simulink model "Virtual_Exhaust_Aftertreatment_Controller_PRT"  (R2016b)
settings: Solver=FixedStepAuto  StartTime=0.0  StopTime=inf  FixedStep=VirtExhATCtrlr.tiSimnTiStep_C  RelTol=1e-3  SampleTimeConstraint=STIndependent  EnableMultiTasking=on
undefined symbols (not defined in the file or in its folder): CAL, SOUIT, T3LIMCL_COEOM_MSK_SY, T3LimCL_stMskEOM1_C, T3LimCL_stMskEOM2_C, T3LimCL_stMskEOM3_C, VirtExhATCtrlr_numHrznSize_CA
libraries: simulink x4
(part 1 of 5)
settings Model: Creator=m01wolf  LastModifiedBy=bunver
settings DataIOCC: SaveFormat=StructureWithTime  SaveOutput=off  DSMLogging=off  VisualizeSimOutput=off  SaveTime=off  StateSaveName=Results  SignalLoggingName=Results
settings OptimizationCC: BlockReduction=off  ConditionallyExecuteInputs=off  LifeSpan=inf
settings DebuggingCC: AllowSymbolicDim=off  SFUnexpectedBacktrackingDiag=warning  SFNoUnconditionalDefaultTransitionDiag=warning  SFExecutionAtInitializationDiag=none
settings ModelReferenceCC: ModelReferenceNumInstancesAllowed=Single  PropagateSignalLabelsOutOfModel=off
settings GRTTargetCC: TargetLangStandard=C89/C90 (ANSI)
settings ConfigComp: CovMetricSettings=dw  CovHtmlReporting=on  CovSaveCumulativeToWorkspaceVar=on  CovSaveSingleToWorkspaceVar=on  CovExternalEMLEnable=off

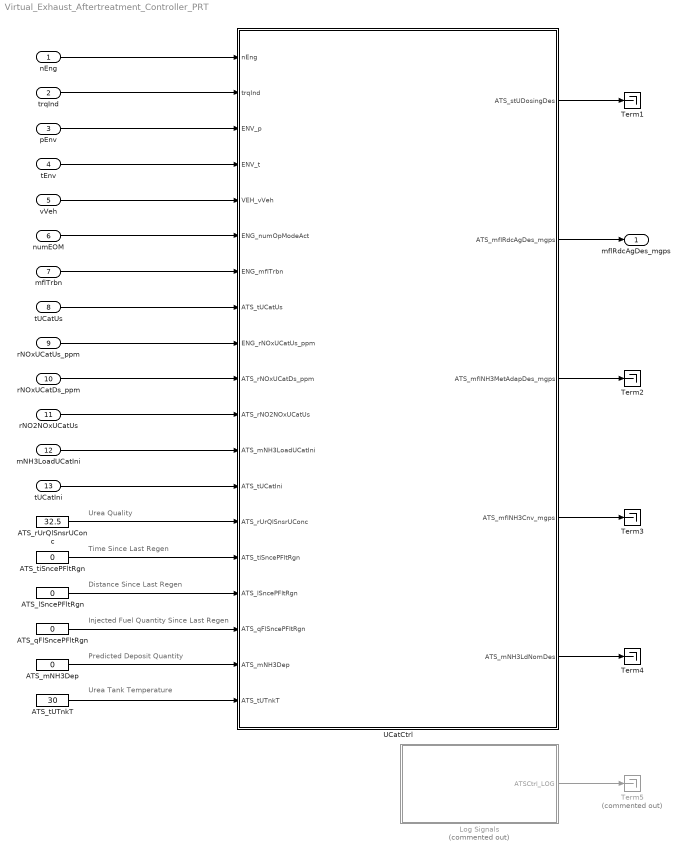
== system Virtual_Exhaust_Aftertreatment_Controller_PRT ==
  note: Urea Quality
  note: Time Since Last Regen
  note: Distance Since Last Regen
  note: Urea Tank Temperature
  note: Predicted Deposit Quantity
  note: Injected Fuel Quantity Since Last Regen
  nEng : Inport  PortDimensions=VirtExhATCtrlr_numHrznSize_CA
  trqInd : Inport  Port=2  PortDimensions=VirtExhATCtrlr_numHrznSize_CA
  "pEnv  " : Inport  Port=3  OutDataTypeStr=double
  "tEnv  " : Inport  Port=4  OutDataTypeStr=double
  vVeh : Inport  Port=5  OutDataTypeStr=double  PortDimensions=VirtExhATCtrlr_numHrznSize_CA
  numEOM : Inport  Port=6  PortDimensions=VirtExhATCtrlr_numHrznSize_CA
  mflTrbn : Inport  Port=7  PortDimensions=VirtExhATCtrlr_numHrznSize_CA
  tUCatUs : Inport  Port=8  PortDimensions=VirtExhATCtrlr_numHrznSize_CA
  rNOxUCatUs_ppm : Inport  Port=9  PortDimensions=VirtExhATCtrlr_numHrznSize_CA
  rNOxUCatDs_ppm : Inport  Port=10  PortDimensions=VirtExhATCtrlr_numHrznSize_CA
  rNO2NOxUCatUs : Inport  Port=11  PortDimensions=VirtExhATCtrlr_numHrznSize_CA
  mNH3LoadUCatIni : Inport  Port=12
  tUCatIni : Inport  Port=13
  ATS_lSncePFltRgn : Constant  Value=0  SampleTime=-1
  ATS_mNH3Dep : Constant  Value=0  SampleTime=-1
  ATS_qFlSncePFltRgn : Constant  Value=0  SampleTime=-1
  ATS_rUrQlSnsrUConc : Constant  Value=32.5  SampleTime=-1
  ATS_tUTnkT : Constant  Value=30  SampleTime=-1
  ATS_tiSncePFltRgn : Constant  Value=0  SampleTime=-1
  Log Signals : Subsystem  Commented=on
  Term{1..4} (4 alike) : Terminator
  Term5 : Terminator  Commented=on
  UCatCtrl : Subsystem
  mflRdcAgDes_mgps : Outport
  wires:
  UCatCtrl/1(ATS_stUDosingDes) -> Term1/1
  UCatCtrl/2(ATS_mflRdcAgDes_mgps) -> mflRdcAgDes_mgps/1
  UCatCtrl/3(ATS_mflNH3MetAdapDes_mgps) -> Term2/1
  UCatCtrl/4(ATS_mflNH3Cnv_mgps) -> Term3/1
  UCatCtrl/5(ATS_mNH3LdNomDes) -> Term4/1
  Log Signals/1(ATSCtrl_LOG) -> Term5/1
  nEng/1 -> UCatCtrl/1(nEng)
  trqInd/1 -> UCatCtrl/2(trqInd)
  "pEnv  "/1 -> UCatCtrl/3(ENV_p)
  "tEnv  "/1 -> UCatCtrl/4(ENV_t)
  vVeh/1 -> UCatCtrl/5(VEH_vVeh)
  numEOM/1 -> UCatCtrl/6(ENG_numOpModeAct)
  mflTrbn/1 -> UCatCtrl/7(ENG_mflTrbn)
  tUCatUs/1 -> UCatCtrl/8(ATS_tUCatUs)
  rNOxUCatUs_ppm/1 -> UCatCtrl/9(ENG_rNOxUCatUs_ppm)
  rNOxUCatDs_ppm/1 -> UCatCtrl/10(ATS_rNOxUCatDs_ppm)
  rNO2NOxUCatUs/1 -> UCatCtrl/11(ATS_rNO2NOxUCatUs)
  mNH3LoadUCatIni/1 -> UCatCtrl/12(ATS_mNH3LoadUCatIni)
  tUCatIni/1 -> UCatCtrl/13(ATS_tUCatIni)
  ATS_tiSncePFltRgn/1 -> UCatCtrl/15(ATS_tiSncePFltRgn)
  ATS_qFlSncePFltRgn/1 -> UCatCtrl/17(ATS_qFlSncePFltRgn)
  ATS_tUTnkT/1 -> UCatCtrl/19(ATS_tUTnkT)
  ATS_mNH3Dep/1 -> UCatCtrl/18(ATS_mNH3Dep)
  ATS_lSncePFltRgn/1 -> UCatCtrl/16(ATS_lSncePFltRgn)
  ATS_rUrQlSnsrUConc/1 -> UCatCtrl/14(ATS_rUrQlSnsrUConc)

== system Virtual_Exhaust_Aftertreatment_Controller_PRT/Log Signals ==
  BusCreator1 : BusCreator  Inputs=23
  ATSCtrl_LOG : Outport
  wires:
  BusCreator1/1 -> ATSCtrl_LOG/1  "ATSCtrl_LOG_BUS"
  [ATS_etaEstNOxCnvUCat] -> BusCreator1/1
  [ATS_facEstEfcUCatAge] -> BusCreator1/2
  [ATS_mEstNH3LoadUCat] -> BusCreator1/3
  [ATS_mflEstNH3OxiUCatUs_mgps] -> BusCreator1/4
  [ATS_rEstNOxUCatDs_ppm] -> BusCreator1/5
  [ATS_tEstUCatAvrg] -> BusCreator1/6
  [ATS_mflNH3OxiUCatUs_mgps] -> BusCreator1/7
  [DepLimCor_facNH3MaxCor] -> BusCreator1/8
  [SCRLdG_dmNH3Max] -> BusCreator1/9
  [ATS_facNOxCtl] -> BusCreator1/10
  [ATS_facQtyAdap] -> BusCreator1/11
  [ATS_mNH3LdNom] -> BusCreator1/12
  [ATS_mNH3LoadUCatRst] -> BusCreator1/13
  [ATS_mflNH3Cnv_mgps] -> BusCreator1/14
  [ATS_mflNH3CurrEfc_mgps] -> BusCreator1/15
  [ATS_mflNH3DpstLmt_mgps] -> BusCreator1/16
  [ATS_mflNH3MetAdapDes_mgps] -> BusCreator1/17
  [ATS_mflNH3PreCtl_mgps] -> BusCreator1/18
  [ATS_mflNH3_mgps] -> BusCreator1/19
  [ATS_mflNOxUs_mgps] -> BusCreator1/20
  [ATS_stNH3LoadUCatRst] -> BusCreator1/21
  [ATS_stUDosing] -> BusCreator1/22
  [EvpMod_tUCatUsT] -> BusCreator1/23

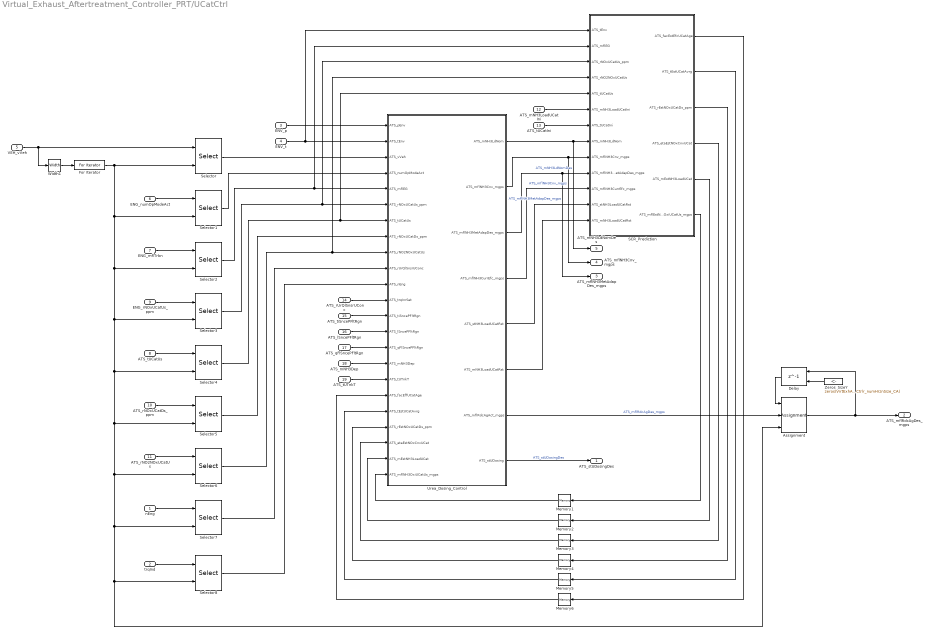
== system Virtual_Exhaust_Aftertreatment_Controller_PRT/UCatCtrl ==
  nEng : Inport
  trqInd : Inport  Port=2
  ENV_p : Inport  Port=3
  ENV_t : Inport  Port=4
  VEH_vVeh : Inport  Port=5
  ENG_numOpModeAct : Inport  Port=6
  ENG_mflTrbn : Inport  Port=7
  ATS_tUCatUs : Inport  Port=8
  ENG_rNOxUCatUs_ppm : Inport  Port=9
  ATS_rNOxUCatDs_ppm : Inport  Port=10
  ATS_rNO2NOxUCatUs : Inport  Port=11
  ATS_mNH3LoadUCatIni : Inport  Port=12
  ATS_tUCatIni : Inport  Port=13
  ATS_rUrQlSnsrUConc : Inport  Port=14
  ATS_tiSncePFltRgn : Inport  Port=15
  ATS_lSncePFltRgn : Inport  Port=16
  ATS_qFlSncePFltRgn : Inport  Port=17
  ATS_mNH3Dep : Inport  Port=18
  ATS_tUTnkT : Inport  Port=19
  Assignment : Assignment  DiagnosticForDimensions=Warning  IndexOptions=Starting index (port)  Indices=1  OutputSizes=1
  Delay : Delay  DelayLength=1  InitialConditionSource=Input port
      settings: InputPortMap=u0,p4
  For Iterator : ForIterator  IterationSource=external  IterationLimit=300
  Memory1 : Memory  InheritSampleTime=on
  Memory2 : Memory  InheritSampleTime=on
  Memory3 : Memory  X0=1  InheritSampleTime=on
  Memory4 : Memory  InheritSampleTime=on
  Memory5 : Memory  X0=100  InheritSampleTime=on
  Memory6 : Memory  X0=1  InheritSampleTime=on
  SCR_Prediction : Subsystem
  Selector{,1..8} (9 alike) : Selector  InputPortWidth=VirtExhATCtrlr_numHrznSize_CA(1)  IndexOptions=Index vector (port)  Indices=[1 3]  OutputSizes=1
  Urea_Dosing_Control : Subsystem
  Width1 : Width
  Zeros_SizeY : Constant  Value=zeros(VirtExhATCtrlr_numHrznSize_CA)
  ATS_stUDosingDes : Outport
  ATS_mflRdcAgDes_mgps : Outport  Port=2
  ATS_mflNH3MetAdapDes_mgps : Outport  Port=3
  ATS_mflNH3Cnv_mgps : Outport  Port=4
  ATS_mNH3LdNomDes : Outport  Port=5
  wires:
  Memory6/1 -> Urea_Dosing_Control/18(ATS_facEffUCatAge)
  Memory4/1 -> Urea_Dosing_Control/20(ATS_rEstNOxUCatDs_ppm)
  Memory3/1 -> Urea_Dosing_Control/21(ATS_etaEstNOxCnvUCat)
  Memory1/1 -> Urea_Dosing_Control/23(ATS_mflNH3OxiUCatUs_mgps)
  SCR_Prediction/1(ATS_facEstEfcUCatAge) -> Memory6/1
  Urea_Dosing_Control/8(ATS_stUDosing) -> ATS_stUDosingDes/1  "ATS_stUDosingDes"
  Urea_Dosing_Control/6(ATS_mNH3LoadUCatRst) -> SCR_Prediction/13(ATS_mNH3LoadUCatRst)
  Urea_Dosing_Control/5(ATS_stNH3LoadUCatRst) -> SCR_Prediction/12(ATS_stNH3LoadUCatRst)
  Urea_Dosing_Control/4(ATS_mflNH3CurrEfc_mgps) -> SCR_Prediction/11(ATS_mflNH3CurrEfc_mgps)
  Urea_Dosing_Control/3(ATS_mflNH3MetAdapDes_mgps) -> SCR_Prediction/10(ATS_mflNH3MetAdapDes_mgps), ATS_mflNH3MetAdapDes_mgps/1  "ATS_mflNH3MetAdapDes_mgps"
  Urea_Dosing_Control/2(ATS_mflNH3Cnv_mgps) -> SCR_Prediction/9(ATS_mflNH3Cnv_mgps), ATS_mflNH3Cnv_mgps/1  "ATS_mflNH3Cnv_mgps"
  Urea_Dosing_Control/1(ATS_mNH3LdNom) -> SCR_Prediction/8(ATS_mNH3LdNom), ATS_mNH3LdNomDes/1  "ATS_mNH3LdNomDes"
  ATS_tUCatIni/1 -> SCR_Prediction/7(ATS_tUCatIni)
  ATS_mNH3LoadUCatIni/1 -> SCR_Prediction/6(ATS_mNH3LoadUCatIni)
  SCR_Prediction/3(ATS_rEstNOxUCatDs_ppm) -> Memory4/1
  SCR_Prediction/4(ATS_etaEstNOxCnvUCat) -> Memory3/1
  SCR_Prediction/6(ATS_mflEstNH3OxiUCatUs_mgps) -> Memory1/1
  ENV_p/1 -> Urea_Dosing_Control/1(ATS_pEnv)
  ENV_t/1 -> SCR_Prediction/1(ATS_tEnv), Urea_Dosing_Control/2(ATS_tEnv)
  VEH_vVeh/1 -> Width1/1, Selector/1
  Selector3/1 -> SCR_Prediction/3(ATS_rNOxUCatUs_ppm), Urea_Dosing_Control/6(ATS_rNOxUCatUs_ppm)
  ATS_tUCatUs/1 -> Selector4/1
  ENG_numOpModeAct/1 -> Selector1/1
  ENG_rNOxUCatUs_ppm/1 -> Selector3/1
  Selector/1 -> Urea_Dosing_Control/3(ATS_vVeh)
  For Iterator/1 -> Selector/2, Selector1/2, Selector2/2, Selector3/2, Selector4/2, Selector5/2, Selector7/2, Selector8/2, Assignment/3, Selector6/2
  Selector2/1 -> SCR_Prediction/2(ATS_mflEG), Urea_Dosing_Control/5(ATS_mflEG)
  Selector4/1 -> SCR_Prediction/5(ATS_tUCatUs), Urea_Dosing_Control/7(ATS_tUCatUs)
  Selector6/1 -> SCR_Prediction/4(ATS_rNO2NOxUCatUs), Urea_Dosing_Control/9(ATS_rNO2NOxUCatUs)
  Width1/1 -> For Iterator/1
  Selector5/1 -> Urea_Dosing_Control/8(ATS_rNOxUCatDs_ppm)
  Selector1/1 -> Urea_Dosing_Control/4(ATS_numOpModeAct)
  Zeros_SizeY/1 -> Delay/2
  Assignment/1 -> Delay/1, ATS_mflRdcAgDes_mgps/1
  SCR_Prediction/5(ATS_mEstNH3LoadUCat) -> Memory2/1
  Memory2/1 -> Urea_Dosing_Control/22(ATS_mEstNH3LoadUCat)
  SCR_Prediction/2(ATS_tEstUCatAvrg) -> Memory5/1
  Memory5/1 -> Urea_Dosing_Control/19("ATS_tEstUCatAvrg ")
  ENG_mflTrbn/1 -> Selector2/1
  ATS_rNOxUCatDs_ppm/1 -> Selector5/1
  ATS_rNO2NOxUCatUs/1 -> Selector6/1
  Urea_Dosing_Control/7(ATS_mflRdcAgAct_mgps) -> Assignment/2  "ATS_mflRdcAgDes_mgps"
  Delay/1 -> Assignment/1
  ATS_rUrQlSnsrUConc/1 -> Urea_Dosing_Control/12(ATS_trqInrSet)
  ATS_tiSncePFltRgn/1 -> Urea_Dosing_Control/13(ATS_tiSncePFltRgn)
  ATS_lSncePFltRgn/1 -> Urea_Dosing_Control/14(ATS_lSncePFltRgn)
  ATS_qFlSncePFltRgn/1 -> Urea_Dosing_Control/15(ATS_qFlSncePFltRgn)
  ATS_mNH3Dep/1 -> Urea_Dosing_Control/16(ATS_mNH3Dep)
  ATS_tUTnkT/1 -> Urea_Dosing_Control/17(ATS_tUTnkT)
  nEng/1 -> Selector7/1
  Selector7/1 -> Urea_Dosing_Control/10(ATS_rUrQlSnsrUConc)
  Selector8/1 -> Urea_Dosing_Control/11(ATS_nEng)
  trqInd/1 -> Selector8/1

== system Virtual_Exhaust_Aftertreatment_Controller_PRT/UCatCtrl/SCR_Prediction ==
  ATS_tEnv : Inport
  ATS_mflEG : Inport  Port=2
  ATS_rNOxUCatUs_ppm : Inport  Port=3
  ATS_rNO2NOxUCatUs : Inport  Port=4
  ATS_tUCatUs : Inport  Port=5
  ATS_mNH3LoadUCatIni : Inport  Port=6
  ATS_tUCatIni : Inport  Port=7
  ATS_mNH3LdNom : Inport  Port=8
  ATS_mflNH3Cnv_mgps : Inport  Port=9
  ATS_mflNH3MetAdapDes_mgps : Inport  Port=10
  ATS_mflNH3CurrEfc_mgps : Inport  Port=11
  ATS_stNH3LoadUCatRst : Inport  Port=12
  ATS_mNH3LoadUCatRst : Inport  Port=13
  GOTO_ATS_etaEstNOxCnvUCat : Subsystem  mask{SIG='ATS_etaEstNOxCnvUCat'}
      mask prompts: SIG "Log Signal Name"
      mask init:
      | lines = find_system(gcb, 'LookUnderMasks', 'on', 'FindAll', 'on', 'Type', 'Line');
      | gotob = find_system(gcb, 'LookUnderMasks', 'on', 'FindAll', 'on', 'Type', 'Block', 'Name', 'GotoXX');
      | inblk = find_system(gcb, 'LookUnderMasks', 'on', 'FindAll', 'on', 'Type', 'Block', 'BlockType', 'Inport');
      | lineS = get(lines,'SourcePort');
      | for i = 1:numel(lineS)
      |     if strcmp(lineS{i}, 'GainXX:1')
      |         set(lines(i), 'Name', SIG);
      |     else %if strcmp(lineS{i}, 'InXX:1')
      |         inName = get(lines(i), 'Name');
      |         if ~isempty(inName)
      |             set(inblk, 'Name', inName);
      |         end
      |     end
      | end
      | set(gotob,'GotoTag', SIG);
      | set(gcbh,'Name', ['GOTO_',SIG]);
      mask Display: fprintf(SIG);
  GOTO_ATS_facEstEfcUCatAge : Subsystem  mask{SIG='ATS_facEstEfcUCatAge'}
      mask prompts: SIG "Log Signal Name"
      mask init: same as Virtual_Exhaust_Aftertreatment_Controller_PRT/UCatCtrl/SCR_Prediction/GOTO_ATS_etaEstNOxCnvUCat
      mask Display: fprintf(SIG);
  GOTO_ATS_mEstNH3LoadUCat : Subsystem  mask{SIG='ATS_mEstNH3LoadUCat'}
      mask prompts: SIG "Log Signal Name"
      mask init: same as Virtual_Exhaust_Aftertreatment_Controller_PRT/UCatCtrl/SCR_Prediction/GOTO_ATS_etaEstNOxCnvUCat
      mask Display: fprintf(SIG);
  GOTO_ATS_mflEstNH3OxiUCatUs_mgps : Subsystem  mask{SIG='ATS_mflEstNH3OxiUCatUs_mgps'}
      mask prompts: SIG "Log Signal Name"
      mask init: same as Virtual_Exhaust_Aftertreatment_Controller_PRT/UCatCtrl/SCR_Prediction/GOTO_ATS_etaEstNOxCnvUCat
      mask Display: fprintf(SIG);
  GOTO_ATS_rEstNOxUCatDs_ppm : Subsystem  mask{SIG='ATS_rEstNOxUCatDs_ppm'}
      mask prompts: SIG "Log Signal Name"
      mask init: same as Virtual_Exhaust_Aftertreatment_Controller_PRT/UCatCtrl/SCR_Prediction/GOTO_ATS_etaEstNOxCnvUCat
      mask Display: fprintf(SIG);
  GOTO_ATS_tEstUCatAvrg : Subsystem  mask{SIG='ATS_tEstUCatAvrg'}
      mask prompts: SIG "Log Signal Name"
      mask init: same as Virtual_Exhaust_Aftertreatment_Controller_PRT/UCatCtrl/SCR_Prediction/GOTO_ATS_etaEstNOxCnvUCat
      mask Display: fprintf(SIG);
  Main : Subsystem
  NOx Downstream Prediction : Subsystem
  ATS_facEstEfcUCatAge : Outport
  ATS_tEstUCatAvrg : Outport  Port=2
  ATS_rEstNOxUCatDs_ppm : Outport  Port=3
  ATS_etaEstNOxCnvUCat : Outport  Port=4
  ATS_mEstNH3LoadUCat : Outport  Port=5
  ATS_mflEstNH3OxiUCatUs_mgps : Outport  Port=6
  wires:
  ATS_mNH3LdNom/1 -> Main/9(ATS_mNH3LdNom)
  ATS_mflNH3Cnv_mgps/1 -> Main/8(ATS_mflNH3Cnv_mgps)
  ATS_mflNH3CurrEfc_mgps/1 -> Main/7(ATS_mflNH3CurrEfc_mgps)
  Main/2(ATS_etaEstNOxCnvUCat) -> ATS_etaEstNOxCnvUCat/1, NOx Downstream Prediction/1(ATS_etaEstNOxCnvUCat), GOTO_ATS_etaEstNOxCnvUCat/1(InXX)
  Main/1(ATS_tEstUCatAvrg) -> ATS_tEstUCatAvrg/1, GOTO_ATS_tEstUCatAvrg/1(InXX)
  Main/3(ATS_mEstNH3LdUCat) -> ATS_mEstNH3LoadUCat/1, GOTO_ATS_mEstNH3LoadUCat/1(InXX)
  ATS_rNOxUCatUs_ppm/1 -> NOx Downstream Prediction/2(ATS_rNOxUCatUs_ppm), Main/3(ATS_rNOxUCatUs_ppm)
  ATS_mflEG/1 -> Main/1(ATS_mflEG)
  ATS_rNO2NOxUCatUs/1 -> Main/2(ATS_rNO2NOxUCatUs)
  ATS_tUCatUs/1 -> Main/6(ATS_tUCatUs)
  ATS_tEnv/1 -> Main/5(ATS_tEnv)
  NOx Downstream Prediction/1("ATS_rEstNOxUCatDs_ppm ") -> GOTO_ATS_rEstNOxUCatDs_ppm/1(InXX), ATS_rEstNOxUCatDs_ppm/1
  Main/4(ATS_mflNH3OxiUCatUs_mgps) -> ATS_mflEstNH3OxiUCatUs_mgps/1, GOTO_ATS_mflEstNH3OxiUCatUs_mgps/1(InXX)
  ATS_stNH3LoadUCatRst/1 -> Main/10(ATS_stNH3LoadUCatRst)
  ATS_mflNH3MetAdapDes_mgps/1 -> Main/11(ATS_mflNH3MetAdapDes_mgps)
  Main/5(ATS_facEstEfcUCatAge) -> ATS_facEstEfcUCatAge/1, GOTO_ATS_facEstEfcUCatAge/1(InXX)
  ATS_mNH3LoadUCatRst/1 -> Main/13(ATS_mNH3LoadUCatRst)
  ATS_mNH3LoadUCatIni/1 -> Main/12(ATS_mNH3LoadUCatIni)
  ATS_tUCatIni/1 -> Main/4(ATS_tUCatIni)

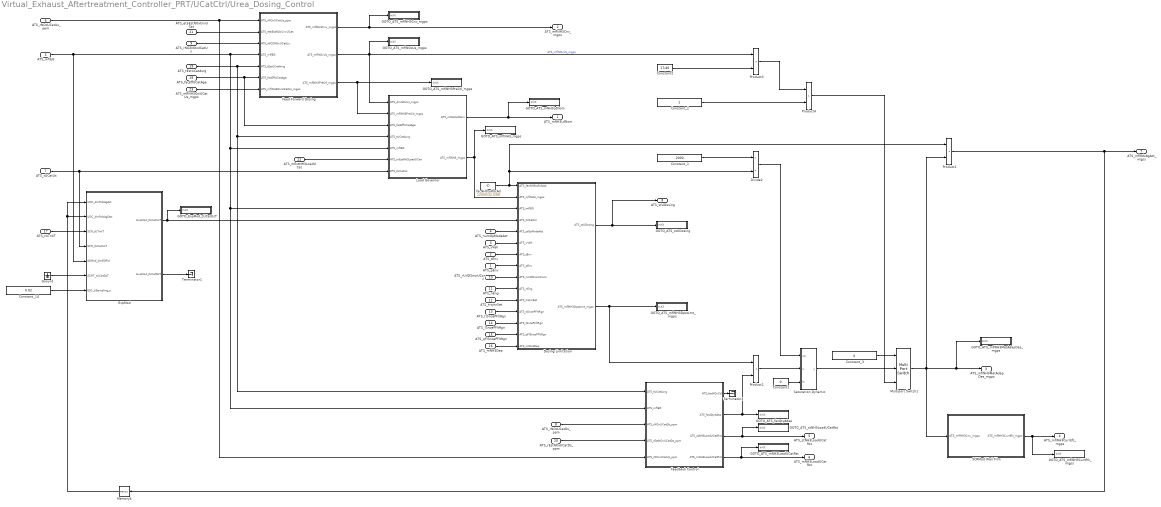
== system Virtual_Exhaust_Aftertreatment_Controller_PRT/UCatCtrl/Urea_Dosing_Control ==
  ATS_pEnv : Inport
  ATS_tEnv : Inport  Port=2
  ATS_vVeh : Inport  Port=3
  ATS_numOpModeAct : Inport  Port=4
  ATS_mflEG : Inport  Port=5
  ATS_rNOxUCatUs_ppm : Inport  Port=6
  ATS_tUCatUs : Inport  Port=7
  ATS_rNOxUCatDs_ppm : Inport  Port=8
  ATS_rNO2NOxUCatUs : Inport  Port=9
  ATS_rUrQlSnsrUConc : Inport  Port=10
  ATS_nEng : Inport  Port=11
  ATS_trqInrSet : Inport  Port=12
  ATS_tiSncePFltRgn : Inport  Port=13
  ATS_lSncePFltRgn : Inport  Port=14
  ATS_qFlSncePFltRgn : Inport  Port=15
  ATS_mNH3Dep : Inport  Port=16
  ATS_tUTnkT : Inport  Port=17
  ATS_facEffUCatAge : Inport  Port=18
  "ATS_tEstUCatAvrg " : Inport  Port=19
  ATS_rEstNOxUCatDs_ppm : Inport  Port=20
  ATS_etaEstNOxCnvUCat : Inport  Port=21
  ATS_mEstNH3LoadUCat : Inport  Port=22
  ATS_mflNH3OxiUCatUs_mgps : Inport  Port=23
  Constant1 : Constant  Value=0  SampleTime=-1
  Constant2 : Constant  Value=17/46  SampleTime=-1
  Constant_1 : Constant  Value=2000  SampleTime=-1
  Constant_14 : Constant  Value=0.02  SampleTime=-1
  Constant_2 : Constant  SampleTime=-1
  Constant_3 : Constant  Value=0  SampleTime=-1
  Divide2 : Product  Inputs=*/
  Dosing Limitation : Subsystem
  EvpMod : Subsystem
  Feed Forward Dosing : Subsystem
  Feedback Control : Subsystem
  GOTO_ATS_facQtyAdap : Subsystem  mask{SIG='ATS_facQtyAdap'}
      mask prompts: SIG "Log Signal Name"
      mask init: same as Virtual_Exhaust_Aftertreatment_Controller_PRT/UCatCtrl/SCR_Prediction/GOTO_ATS_etaEstNOxCnvUCat
      mask Display: fprintf(SIG);
  GOTO_ATS_mNH3LdNom : Subsystem  mask{SIG='ATS_mNH3LdNom'}
      mask prompts: SIG "Log Signal Name"
      mask init: same as Virtual_Exhaust_Aftertreatment_Controller_PRT/UCatCtrl/SCR_Prediction/GOTO_ATS_etaEstNOxCnvUCat
      mask Display: fprintf(SIG);
  GOTO_ATS_mNH3LoadUCatRst : Subsystem  mask{SIG='ATS_mNH3LoadUCatRst'}
      mask prompts: SIG "Log Signal Name"
      mask init: same as Virtual_Exhaust_Aftertreatment_Controller_PRT/UCatCtrl/SCR_Prediction/GOTO_ATS_etaEstNOxCnvUCat
      mask Display: fprintf(SIG);
  GOTO_ATS_mflNH3Cnv_mgps : Subsystem  mask{SIG='ATS_mflNH3Cnv_mgps'}
      mask prompts: SIG "Log Signal Name"
      mask init: same as Virtual_Exhaust_Aftertreatment_Controller_PRT/UCatCtrl/SCR_Prediction/GOTO_ATS_etaEstNOxCnvUCat
      mask Display: fprintf(SIG);
  GOTO_ATS_mflNH3CurrEfc_mgps : Subsystem  mask{SIG='ATS_mflNH3CurrEfc_mgps'}
      mask prompts: SIG "Log Signal Name"
      mask init: same as Virtual_Exhaust_Aftertreatment_Controller_PRT/UCatCtrl/SCR_Prediction/GOTO_ATS_etaEstNOxCnvUCat
      mask Display: fprintf(SIG);
  GOTO_ATS_mflNH3DpstLmt_mgps : Subsystem  mask{SIG='ATS_mflNH3DpstLmt_mgps'}
      mask prompts: SIG "Log Signal Name"
      mask init: same as Virtual_Exhaust_Aftertreatment_Controller_PRT/UCatCtrl/SCR_Prediction/GOTO_ATS_etaEstNOxCnvUCat
      mask Display: fprintf(SIG);
  GOTO_ATS_mflNH3MetAdapDes_mgps : Subsystem  mask{SIG='ATS_mflNH3MetAdapDes_mgps'}
      mask prompts: SIG "Log Signal Name"
      mask init: same as Virtual_Exhaust_Aftertreatment_Controller_PRT/UCatCtrl/SCR_Prediction/GOTO_ATS_etaEstNOxCnvUCat
      mask Display: fprintf(SIG);
  GOTO_ATS_mflNH3PreCtl_mgps : Subsystem  mask{SIG='ATS_mflNH3PreCtl_mgps'}
      mask prompts: SIG "Log Signal Name"
      mask init: same as Virtual_Exhaust_Aftertreatment_Controller_PRT/UCatCtrl/SCR_Prediction/GOTO_ATS_etaEstNOxCnvUCat
      mask Display: fprintf(SIG);
  GOTO_ATS_mflNH3_mgps : Subsystem  mask{SIG='ATS_mflNH3_mgps'}
      mask prompts: SIG "Log Signal Name"
      mask init: same as Virtual_Exhaust_Aftertreatment_Controller_PRT/UCatCtrl/SCR_Prediction/GOTO_ATS_etaEstNOxCnvUCat
      mask Display: fprintf(SIG);
  GOTO_ATS_mflNOxUs_mgps : Subsystem  mask{SIG='ATS_mflNOxUs_mgps'}
      mask prompts: SIG "Log Signal Name"
      mask init: same as Virtual_Exhaust_Aftertreatment_Controller_PRT/UCatCtrl/SCR_Prediction/GOTO_ATS_etaEstNOxCnvUCat
      mask Display: fprintf(SIG);
  GOTO_ATS_stNH3LoadUCatRst : Subsystem  mask{SIG='ATS_stNH3LoadUCatRst'}
      mask prompts: SIG "Log Signal Name"
      mask init: same as Virtual_Exhaust_Aftertreatment_Controller_PRT/UCatCtrl/SCR_Prediction/GOTO_ATS_etaEstNOxCnvUCat
      mask Display: fprintf(SIG);
  GOTO_ATS_stUDosing : Subsystem  mask{SIG='ATS_stUDosing'}
      mask prompts: SIG "Log Signal Name"
      mask init: same as Virtual_Exhaust_Aftertreatment_Controller_PRT/UCatCtrl/SCR_Prediction/GOTO_ATS_etaEstNOxCnvUCat
      mask Display: fprintf(SIG);
  GOTO_EvpMod_tUCatUsT : Subsystem  mask{SIG='EvpMod_tUCatUsT'}
      mask prompts: SIG "Log Signal Name"
      mask init: same as Virtual_Exhaust_Aftertreatment_Controller_PRT/UCatCtrl/SCR_Prediction/GOTO_ATS_etaEstNOxCnvUCat
      mask Display: fprintf(SIG);
  Ground : Ground
  Load Governor : Subsystem
  Memory4 : Memory  InheritSampleTime=on
  Multiport Switch1 : MultiPortSwitch  DataPortOrder=Zero-based contiguous  Inputs=2
  Product{1..4} (4 alike) : Product  RndMeth=Zero
  SCRMod Wall Film : Subsystem
  Saturation Dynamic : Subsystem  mask(Saturation Dynamic){OutMin=[], OutMax=[], OutDataTypeStr=Inherit: Same as second input, OutputDataTypeScalingMode=Same as second input, OutDataType=fixdt(1, 16), OutScaling=2^-10, LockScale=off, RndMeth=Floor, DoSatur=off}
      mask prompts: OutMin "Simulink:masks:OutputMinimum_MP"; OutMax "Simulink:masks:OutputMaximum_MP"; OutDataTypeStr "Simulink:masks:OutputDataType_MP"; OutputDataTypeScalingMode "Simulink:masks:OutputDataTypeMode_MP"; OutDataType "Simulink:masks:OutputDataTypeegFixdt116Fixdtsingle_MP"; OutScaling "Simulink:masks:OutputScalingSlopeEg29OrSlopeBias_MP"; LockScale "Simulink:masks:LockOutputDataTypeAgainstFxpTools_MP"; RndMeth "Simulink:masks:IntegerRoundingMode_MP"; DoSatur "Simulink:masks:SaturateOnIntegerOverflow_MP"
      mask help: Simulink:masks:SaturationDynamic_MD
      mask init:
      | blkH = gcbh;
      | blkName = getfullname(blkH);
      | 
      | switch_blks = {'Switch','Switch2'}; 
      | for i = 1:length(switch_blks)
      |   set_param([blkName,'/',switch_blks{i}], ...
      |       'RndMeth', RndMeth, ...
      | 	  'DoSatur', DoSatur);
      | end
      | 
      | propBlk = [blkName, '/Data Type Propagation'];
      | 
      | if strcmp(OutputDataTypeScalingMode, 'Same as second input')
      |     set_param(propBlk, 'PropDataTypeMode', 'Inherit via propagation rule', ...
      |                        'PropScalingMode',  'Inherit via propagation rule');
      | else
      |     scaling = OutScaling;
      |     scalingMode = 'Specify via dialog';
      |     switch OutputDataTypeScalingMode
      |       case 'double'
      |         dataType = 'fixdt(''double'')';
      |       case 'single'
      |         dataType = 'fixdt(''single'')';
      |       case 'int8'
      |         dataType = 'fixdt(1,8,0)';
      |       case 'uint8'
      |         dataType = 'fixdt(0,8,0)';
      |       case 'int16'
      |         dataType = 'fixdt(1,16,0)';
      |       case 'uint16'
      |         dataType = 'fixdt(0,16,0)';
      |       case 'int32'
      |         dataType = 'fixdt(1,32,0)';
      |       case 'uint32'
      |         dataType = 'fixdt(0,32,0)';
      |       case 'Specify via dialog'
      |         dataType = OutDataType;
      |         if ~isempty(OutDataTypeStr) && isa(OutDataTypeStr,'Simulink.NumericType') 
      |           if strcmp(OutDataTypeStr.DataTypeMode, 'Fixed-point: unspecified scaling') 
      |             scalingMode = 'Obtain via best precision';
      |             range = [OutMin OutMax];
      |             range = range(~isinf(range));
      |             set_param(propBlk, 'ValuesUsedBestPrec', mat2str(range));
      |           end
      |         end
      |     end
      |     
      |     set_param(propBlk, 'PropDataTypeMode', 'Specify via dialog', ...
      |                        'PropScalingMode',  scalingMode, ...
      |                        'PropDataType',     dataType, ...
      |                        'PropScaling',      scaling);
      | end
      mask Callback OutDataTypeStr: fixptdialog(gcbh)
      mask TypeOptions OutputDataTypeScalingMode: double | single | int8 | uint8 | int16 | uint16 | int32 | uint32 | Specify via dialog | Same as second input
      mask Callback OutputDataTypeScalingMode: fixptdialog(gcbh)
      mask Callback OutDataType: fixptdialog(gcbh)
      mask TypeOptions RndMeth: Simulink:masks:Ceiling | Simulink:masks:Convergent | Simulink:masks:Floor | Simulink:masks:Nearest | Simulink:masks:Round | Simulink:masks:Simplest | Simulink:masks:Zero
      mask Display: plot([0.15 0.85],[.5 .5],[.5 .5],[0.05 0.95],0.15+0.7*[0 .25 .75 1],0.05+0.9*[.25 .25 .75 .75]);
  Terminator1 : Terminator
  Terminator3 : Terminator
  facNH3toRdcAd : Constant  Value=12000/32.5/68  SampleTime=-1
  ATS_mNH3LdNom : Outport
  ATS_mflNH3Cnv_mgps : Outport  Port=2
  ATS_mflNH3MetAdapDes_mgps : Outport  Port=3
  ATS_mflNH3CurrEfc_mgps : Outport  Port=4
  ATS_stNH3LoadUCatRst : Outport  Port=5
  ATS_mNH3LoadUCatRst : Outport  Port=6
  ATS_mflRdcAgAct_mgps : Outport  Port=7
  ATS_stUDosing : Outport  Port=8
  wires:
  ATS_facEffUCatAge/1 -> Load Governor/3(ATS_facEffUCatAge), Feed Forward Dosing/6(ATS_facEffUCatAge)
  Feed Forward Dosing/3(ATS_mflNH3PreCtl_mgps) -> GOTO_ATS_mflNH3PreCtl_mgps/1(InXX), Load Governor/2(ATS_mflNH3PreCtl_mgps)
  ATS_mflEG/1 -> Feedback Control/2(ATS_mflEG), Dosing Limitation/3(ATS_mflEG), Load Governor/5(ATS_mflEG), Feed Forward Dosing/4(ATS_mflEG), EvpMod/5(ASMod_dmEGFld)
  ATS_rNO2NOxUCatUs/1 -> Feed Forward Dosing/3(ATS_rNO2NOxUCatUs)
  ATS_rNOxUCatUs_ppm/1 -> Feedback Control/5(ATS_rNOxUCatUs_ppm), Feed Forward Dosing/1(ATS_rNOxUCatUs_ppm)
  "ATS_tEstUCatAvrg "/1 -> Feed Forward Dosing/5(ATS_tEstUCatAvrg), Load Governor/4(ATS_tUCatAvrg), Feedback Control/1("ATS_tUCatAvrg ")
  Load Governor/2(ATS_mflNH3_mgps) -> GOTO_ATS_mflNH3_mgps/1(InXX), Dosing Limitation/2(ATS_mflNH3_mgps)
  ATS_tUCatUs/1 -> EvpMod/4(SCR_tUCatUsT), Load Governor/7(ATS_tUCatUs)
  ATS_etaEstNOxCnvUCat/1 -> Feed Forward Dosing/2(ATS_etaEstNOxCnvUCat)
  ATS_mEstNH3LoadUCat/1 -> Load Governor/6(ATS_mEstNH3LoadUCat)
  Feed Forward Dosing/1(ATS_mflNH3Cnv_mgps) -> GOTO_ATS_mflNH3Cnv_mgps/1(InXX), ATS_mflNH3Cnv_mgps/1
  Load Governor/1(ATS_mNH3LdNom) -> GOTO_ATS_mNH3LdNom/1(InXX), ATS_mNH3LdNom/1
  Dosing Limitation/2(ATS_mflNH3DpstLmt_mgps) -> GOTO_ATS_mflNH3DpstLmt_mgps/1(InXX), Product2/1
  ATS_rNOxUCatDs_ppm/1 -> Feedback Control/3("ATS_rNOxUCatDs_ppm ")
  Feedback Control/2(ATS_facQtyAdap) -> GOTO_ATS_facQtyAdap/1(InXX), Product2/2
  Product2/1 -> Saturation Dynamic/2(u)
  ATS_rEstNOxUCatDs_ppm/1 -> Feedback Control/4(ATS_rEstNOxUCatDs_ppm)
  Feedback Control/1(ATS_facNOxCtl) -> Terminator3/1
  Feed Forward Dosing/2(ATS_mflNOxUs_mgps) -> GOTO_ATS_mflNOxUs_mgps/1(InXX), Load Governor/1(ATS_dmNOxUs_mgps), Product3/1  "ATS_mflNOxUs_mgps"
  Constant_1/1 -> Divide2/1
  Divide2/1 -> Saturation Dynamic/1(up)
  Constant1/1 -> Saturation Dynamic/3(lo)
  SCRMod Wall Film/1(ATS_mflNH3CurrEfc_mgps) -> GOTO_ATS_mflNH3CurrEfc_mgps/1(InXX), ATS_mflNH3CurrEfc_mgps/1
  ATS_mflNH3OxiUCatUs_mgps/1 -> Feed Forward Dosing/7(ATS_mflNH3OxiUCatUs_mgps)
  Feedback Control/3(ATS_stNH3LoadUCatRst) -> GOTO_ATS_stNH3LoadUCatRst/1(InXX), ATS_stNH3LoadUCatRst/1
  Feedback Control/4(ATS_mNH3LoadUCatRst) -> GOTO_ATS_mNH3LoadUCatRst/1(InXX), ATS_mNH3LoadUCatRst/1
  Multiport Switch1/1 -> SCRMod Wall Film/1(ATS_mflNH3Cnv_mgps), Product1/2, GOTO_ATS_mflNH3MetAdapDes_mgps/1(InXX), ATS_mflNH3MetAdapDes_mgps/1
  facNH3toRdcAd/1 -> Product1/1, Divide2/2, Dosing Limitation/1(ATS_facNH3toRdcAd)
  Product1/1 -> ATS_mflRdcAgAct_mgps/1, Memory4/1
  Dosing Limitation/1(ATS_stUDosing) -> GOTO_ATS_stUDosing/1(InXX), ATS_stUDosing/1
  Constant2/1 -> Product3/2
  Constant_3/1 -> Multiport Switch1/1
  Product3/1 -> Product4/1
  Constant_2/1 -> Product4/2
  Product4/1 -> Multiport Switch1/3
  Saturation Dynamic/1(y) -> Multiport Switch1/2
  ATS_pEnv/1 -> Dosing Limitation/8(ATS_pEnv)
  ATS_tEnv/1 -> Dosing Limitation/7(ATS_tEnv)
  ATS_vVeh/1 -> Dosing Limitation/6(ATS_vVeh)
  ATS_numOpModeAct/1 -> Dosing Limitation/5(ATS_stOpModeAct)
  ATS_mNH3Dep/1 -> Dosing Limitation/15(ATS_mNH3Dep)
  ATS_trqInrSet/1 -> Dosing Limitation/11(ATS_trqInrSet)
  ATS_rUrQlSnsrUConc/1 -> Dosing Limitation/9(ATS_rUrQlSnsrUConc)
  ATS_nEng/1 -> Dosing Limitation/10(ATS_nEng)
  ATS_tiSncePFltRgn/1 -> Dosing Limitation/12(ATS_tiSncePFltRgn)
  ATS_qFlSncePFltRgn/1 -> Dosing Limitation/14(ATS_qFlSncePFltRgn)
  ATS_lSncePFltRgn/1 -> Dosing Limitation/13(ATS_lSncePFltRgn)
  Ground/1 -> EvpMod/6(SCRT_tUCatDsT)
  ATS_tUTnkT/1 -> EvpMod/3(SCR_tUTnkT)
  Constant_14/1 -> EvpMod/7(ESC_tiSampling_s)
  Memory4/1 -> EvpMod/2(UDC_dmRdcAgDes), EvpMod/1(UDC_dmRdcAgAct)
  EvpMod/1(EvpMod_tUCatUsT) -> GOTO_EvpMod_tUCatUsT/1(InXX), Dosing Limitation/4(ATS_tUCatUs)
  EvpMod/2(EvpMod_tUCatDsT) -> Terminator1/1

== system Virtual_Exhaust_Aftertreatment_Controller_PRT/UCatCtrl/SCR_Prediction/GOTO_ATS_etaEstNOxCnvUCat ==
  InXX : Inport
  GainXX : Subsystem
  tag scope: ATS_etaEstNOxCnvUCat=global
  wires:
  GainXX/1(Out) -> [ATS_etaEstNOxCnvUCat]  "ATS_etaEstNOxCnvUCat"
  InXX/1 -> GainXX/1(In)

== system Virtual_Exhaust_Aftertreatment_Controller_PRT/UCatCtrl/SCR_Prediction/GOTO_ATS_facEstEfcUCatAge ==
  InXX : Inport
  GainXX : Subsystem
  tag scope: ATS_facEstEfcUCatAge=global
  wires:
  InXX/1 -> GainXX/1(In)
  GainXX/1(Out) -> [ATS_facEstEfcUCatAge]  "ATS_facEstEfcUCatAge"

== system Virtual_Exhaust_Aftertreatment_Controller_PRT/UCatCtrl/SCR_Prediction/GOTO_ATS_mEstNH3LoadUCat ==
  InXX : Inport
  GainXX : Subsystem
  tag scope: ATS_mEstNH3LoadUCat=global
  wires:
  InXX/1 -> GainXX/1(In)
  GainXX/1(Out) -> [ATS_mEstNH3LoadUCat]  "ATS_mEstNH3LoadUCat"

== system Virtual_Exhaust_Aftertreatment_Controller_PRT/UCatCtrl/SCR_Prediction/GOTO_ATS_mflEstNH3OxiUCatUs_mgps ==
  InXX : Inport
  GainXX : Subsystem
  tag scope: ATS_mflEstNH3OxiUCatUs_mgps=global
  wires:
  GainXX/1(Out) -> [ATS_mflEstNH3OxiUCatUs_mgps]  "ATS_mflEstNH3OxiUCatUs_mgps"
  InXX/1 -> GainXX/1(In)

== system Virtual_Exhaust_Aftertreatment_Controller_PRT/UCatCtrl/SCR_Prediction/GOTO_ATS_rEstNOxUCatDs_ppm ==
  InXX : Inport
  GainXX : Subsystem
  tag scope: ATS_rEstNOxUCatDs_ppm=global
  wires:
  GainXX/1(Out) -> [ATS_rEstNOxUCatDs_ppm]  "ATS_rEstNOxUCatDs_ppm"
  InXX/1 -> GainXX/1(In)

== system Virtual_Exhaust_Aftertreatment_Controller_PRT/UCatCtrl/SCR_Prediction/GOTO_ATS_tEstUCatAvrg ==
  InXX : Inport
  GainXX : Subsystem
  tag scope: ATS_tEstUCatAvrg=global
  wires:
  InXX/1 -> GainXX/1(In)
  GainXX/1(Out) -> [ATS_tEstUCatAvrg]  "ATS_tEstUCatAvrg"

== system Virtual_Exhaust_Aftertreatment_Controller_PRT/UCatCtrl/SCR_Prediction/Main ==
  ATS_mflEG : Inport
  ATS_rNO2NOxUCatUs : Inport  Port=2
  ATS_rNOxUCatUs_ppm : Inport  Port=3
  ATS_tUCatIni : Inport  Port=4
  ATS_tEnv : Inport  Port=5
  ATS_tUCatUs : Inport  Port=6
  ATS_mflNH3CurrEfc_mgps : Inport  Port=7
  ATS_mflNH3Cnv_mgps : Inport  Port=8
  ATS_mNH3LdNom : Inport  Port=9
  ATS_stNH3LoadUCatRst : Inport  Port=10
  ATS_mflNH3MetAdapDes_mgps : Inport  Port=11
  ATS_mNH3LoadUCatIni : Inport  Port=12
  ATS_mNH3LoadUCatRst : Inport  Port=13
  Aging Prediction : Subsystem
  Constant1 : Constant  SampleTime=-1
  Delay2 : Delay  DelayLength=1  InitialConditionSource=Input port  InitialCondition=0
      settings: InputPortMap=u0,p4
  Delay3 : Delay  DelayLength=1  InitialConditionSource=Input port  InitialCondition=0
      settings: InputPortMap=u0,p4
  Term_1 : Terminator
  Term_3 : Terminator
  UCat Efficiency Prediction : Subsystem
  UCat NH3 Load Prediction : Subsystem
  UCat Temperature Prediction : Subsystem
  ATS_tEstUCatAvrg : Outport
  ATS_etaEstNOxCnvUCat : Outport  Port=2
  ATS_mEstNH3LdUCat : Outport  Port=3
  ATS_mflNH3OxiUCatUs_mgps : Outport  Port=4
  ATS_facEstEfcUCatAge : Outport  Port=5
  wires:
  Delay2/1 -> Aging Prediction/1(ATS_tAvrg), ATS_tEstUCatAvrg/1, UCat NH3 Load Prediction/1(ATS_tEstUCatAvrg), UCat Efficiency Prediction/8(ATS_tEstUCatAvrg)
  Delay3/1 -> UCat Efficiency Prediction/3(ATS_facEffUCatAge), UCat NH3 Load Prediction/3(ATS_facEffUCatAge)
  ATS_mNH3LdNom/1 -> UCat Efficiency Prediction/2(SCRLdG_mNH3LdNom)
  UCat Temperature Prediction/1(ATS_tEstUCatAvrg) -> Delay2/1
  UCat Temperature Prediction/3(ATS_tEstUCatFld) -> Term_3/1
  ATS_mflEG/1 -> UCat Temperature Prediction/1(ATS_mflEG), UCat NH3 Load Prediction/2(ATS_mflEG), UCat Efficiency Prediction/4(ATS_mflEG)
  ATS_rNO2NOxUCatUs/1 -> UCat Efficiency Prediction/5(ATS_rNO2NOxUCatUs)
  ATS_rNOxUCatUs_ppm/1 -> UCat Efficiency Prediction/6(ATS_rNOxUCatUs_ppm)
  UCat Temperature Prediction/2(ATS_tEstUCatDs) -> Term_1/1
  ATS_tUCatIni/1 -> UCat Temperature Prediction/4(ATS_tWallUCatIni), Delay2/2
  ATS_tEnv/1 -> UCat Temperature Prediction/3(ATS_tEnv)
  ATS_tUCatUs/1 -> UCat Temperature Prediction/2(ATS_tUCatUs)
  ATS_mflNH3Cnv_mgps/1 -> UCat NH3 Load Prediction/5(ATS_mflNH3Cnv_mgps), UCat Efficiency Prediction/7(ATS_mflNH3Cnv_mgs)
  ATS_mflNH3CurrEfc_mgps/1 -> UCat NH3 Load Prediction/4(ATS_mflNH3CurrEfc_mgps)
  UCat Efficiency Prediction/1(ATS_etaEstNOxCnvUCat) -> ATS_etaEstNOxCnvUCat/1
  UCat NH3 Load Prediction/1(ATS_mflNH3OxiUCatUs_mgps) -> ATS_mflNH3OxiUCatUs_mgps/1
  ATS_stNH3LoadUCatRst/1 -> UCat NH3 Load Prediction/6(ATS_stNH3LoadUCatRst)
  ATS_mflNH3MetAdapDes_mgps/1 -> UCat NH3 Load Prediction/7(ATS_mflNH3MetAdapDes_mgps)
  ATS_mNH3LoadUCatIni/1 -> UCat NH3 Load Prediction/9(ATS_mNH3LoadUCatIni)
  ATS_mNH3LoadUCatRst/1 -> UCat NH3 Load Prediction/8(ATS_mNH3LoadUCatRst)
  Aging Prediction/1(ATS_facEstEfcUCatAge) -> ATS_facEstEfcUCatAge/1, Delay3/1
  Constant1/1 -> Delay3/2
  UCat NH3 Load Prediction/2(ATS_mEstNH3LdUCat) -> UCat Efficiency Prediction/1(ATS_mEstNH3LdUCat), ATS_mEstNH3LdUCat/1

== system Virtual_Exhaust_Aftertreatment_Controller_PRT/UCatCtrl/SCR_Prediction/NOx Downstream Prediction ==
  ATS_etaEstNOxCnvUCat : Inport
  ATS_rNOxUCatUs_ppm : Inport  Port=2
  Product2 : Product  RndMeth=Zero
  Subtract : Sum  Inputs=+-
  constant : Constant  SampleTime=-1
  "ATS_rEstNOxUCatDs_ppm " : Outport
  wires:
  constant/1 -> Subtract/1
  ATS_etaEstNOxCnvUCat/1 -> Subtract/2
  Subtract/1 -> Product2/2
  ATS_rNOxUCatUs_ppm/1 -> Product2/1
  Product2/1 -> "ATS_rEstNOxUCatDs_ppm "/1

== system Virtual_Exhaust_Aftertreatment_Controller_PRT/UCatCtrl/Urea_Dosing_Control/Dosing Limitation ==
  ATS_facNH3toRdcAd : Inport
  ATS_mflNH3_mgps : Inport  Port=2
  ATS_mflEG : Inport  Port=3
  ATS_tUCatUs : Inport  Port=4
  ATS_stOpModeAct : Inport  Port=5
  ATS_vVeh : Inport  Port=6
  ATS_tEnv : Inport  Port=7
  ATS_pEnv : Inport  Port=8
  ATS_rUrQlSnsrUConc : Inport  Port=9
  ATS_nEng : Inport  Port=10
  ATS_trqInrSet : Inport  Port=11
  ATS_tiSncePFltRgn : Inport  Port=12
  ATS_lSncePFltRgn : Inport  Port=13
  ATS_qFlSncePFltRgn : Inport  Port=14
  ATS_mNH3Dep : Inport  Port=15
  Constant1 : Constant  Value=0  SampleTime=-1
  Constant_1 : Constant  SampleTime=-1
  Constant_15 : Constant  Value=0.02  SampleTime=-1
  DepLimCor : Subsystem
  Divide1 : Product  Inputs=*/
  GOTO_DepLimCor_facNH3MaxCor : Subsystem  mask{SIG='DepLimCor_facNH3MaxCor'}
      mask prompts: SIG "Log Signal Name"
      mask init: same as Virtual_Exhaust_Aftertreatment_Controller_PRT/UCatCtrl/SCR_Prediction/GOTO_ATS_etaEstNOxCnvUCat
      mask Display: fprintf(SIG);
  GOTO_SCRLdG_dmNH3Max : Subsystem  mask{SIG='SCRLdG_dmNH3Max'}
      mask prompts: SIG "Log Signal Name"
      mask init: same as Virtual_Exhaust_Aftertreatment_Controller_PRT/UCatCtrl/SCR_Prediction/GOTO_ATS_etaEstNOxCnvUCat
      mask Display: fprintf(SIG);
  Lookup_n-D_3 : Lookup_n-D  BreakpointsForDimension1=[100;150;180;200;225;250;275;300;350;400;500;600;800;1000;1200;1400]  BreakpointsForDimension2=[158.96 159.96 179.96 189.96 199.96 209.96 219.96 229.96 239.96 249.96 259.96 269.96 279.96 299.96 319.96 339.96]  Table=[1.8 1.9 2.25 2.3 4.1 4.6 5.65 8.2 10.2 23.9 31.25 48.45 65.7 143.75 205.35 292;2.7 2.85 3.35 3.45 6.15 6.9 8.45 12.3 14.9 17.9 30.3 58.95 78.9 182.6 228.35 365;3.2 3.4 4.05 4.15 7.35 8.3 10.15 14.75 15.6 21.5 37.75 94.7 108.65 205.9 242.1 365;3.6 3.8 4.5 4.6 8.2 9.2 11.25 16.35 19.7 26.3 55.6 108.65 122.65 221.5 251.35 365;4.05 4.25 5.05 5.2 9.2 10.35 12.65 18.4 21.6 29.55 69.5 126.15 140.2 240.9 262.8 365;4.5 4.75 5.6 5.75 10.25 11.5 14.05 20.45 22.3 32.85 77.2 139.65 157.7 270.1 284.7 365;4.9 5.2 6.2 6.35 11.25 12.65 15.45 22.5 24.6 36.15 85 153.15 175.2 299.3 306.6 365;5.35 5.7 6.75 6.9 12.3 13.8 16.9 24.55 30.5 50.1 92.7 166.6 181.95 328.5 328.5 365;6.25 6.6 7.85 8.05 14.3 16.1 19.7 24 32 70.15 98.3 178.15 195.4 328.5 328.5 365;7.15 7.55 9 9.2 16.35 18.4 22.5 27 35 80.2 112.3 189.7 208.9 328.5 328.5 365;8.95 9.45 11.3 11.5 17 23 23.5 34.5 50 122.5 167.65 212.85 235.85 328.5 328.5 365;10.75 11.35 13.55 13.8 18 27.6 33.75 46.7 75 153.1 194.55 236 328.5 328.5 365 365;14.3 15.15 18 18.4 19 36.85 37.5 57.5 110 153 217.65 282.25 328.5 365 365 365;17.9 18.95 18.95 19 20 46.05 48 60 125 153 240.75 328.5 328.5 365 365 365;21 22 23 24 25 64.45 66 90 175 198 263.25 328.5 328.5 365 365 365;25.05 26.5 31.5 32.25 50 75 90 114.6 250 328.5 365 365 365 365 365 365]  ExtrapMethod=Clip  UseLastTableValue=on  RndMeth=Simplest  InputSameDT=on
  MinMax : MinMax  Inputs=2
  Multiport Switch : MultiPortSwitch  DataPortOrder=Zero-based contiguous  Inputs=2
  Multiport Switch1 : MultiPortSwitch  DataPortOrder=Zero-based contiguous  Inputs=2
  Product1 : Product  RndMeth=Zero
  Product2 : Product  RndMeth=Zero
  Relay_1 : Relay  OnSwitchValue=204.96  OffSwitchValue=184.96
  ATS_stUDosing : Outport
  ATS_mflNH3DpstLmt_mgps : Outport  Port=2
  wires:
  Constant1/1 -> Multiport Switch1/2
  ATS_facNH3toRdcAd/1 -> Divide1/2, Product2/2
  Relay_1/1 -> ATS_stUDosing/1, Multiport Switch1/1
  Multiport Switch/1 -> Product2/1
  ATS_mflNH3_mgps/1 -> Multiport Switch1/3
  Product2/1 -> Divide1/1
  ATS_mflEG/1 -> Lookup_n-D_3/1
  ATS_tUCatUs/1 -> Relay_1/1, DepLimCor/1(SCR_tUCatUsT), Lookup_n-D_3/2
  Product1/1 -> GOTO_SCRLdG_dmNH3Max/1(InXX), MinMax/2
  Divide1/1 -> ATS_mflNH3DpstLmt_mgps/1
  Lookup_n-D_3/1 -> Product1/2
  DepLimCor/1(DepLimCor_facNH3MaxCor) -> GOTO_DepLimCor_facNH3MaxCor/1(InXX), Product1/1
  Constant_1/1 -> Multiport Switch/1
  Multiport Switch1/1 -> Multiport Switch/2, MinMax/1
  MinMax/1 -> Multiport Switch/3
  ATS_pEnv/1 -> DepLimCor/3(EnvP_p)
  ATS_tEnv/1 -> DepLimCor/2(EnvT_t)
  ATS_vVeh/1 -> DepLimCor/4(VehV_v)
  ATS_stOpModeAct/1 -> DepLimCor/10(stOpModeAct)
  ATS_rUrQlSnsrUConc/1 -> DepLimCor/11(UrQlSnsr_ratConc)
  ATS_nEng/1 -> DepLimCor/12(Epm_nEng)
  ATS_trqInrSet/1 -> DepLimCor/13(PthSet_trqInrSet)
  ATS_mNH3Dep/1 -> DepLimCor/9(DepMod_mNH3Dep_mp)
  ATS_tiSncePFltRgn/1 -> DepLimCor/5(PFltRgn_tiSnceRgn)
  ATS_lSncePFltRgn/1 -> DepLimCor/6(PFltRgn_lSnceRgn)
  ATS_qFlSncePFltRgn/1 -> DepLimCor/7(PFltRgn_qFlSnceRgn)
  Constant_15/1 -> DepLimCor/8(ESC_tiSampling_s)

== system Virtual_Exhaust_Aftertreatment_Controller_PRT/UCatCtrl/Urea_Dosing_Control/EvpMod ==
  UDC_dmRdcAgAct : Inport
  UDC_dmRdcAgDes : Inport  Port=2
  SCR_tUTnkT : Inport  Port=3
  SCR_tUCatUsT : Inport  Port=4
  ASMod_dmEGFld : Inport  Port=5
  SCRT_tUCatDsT : Inport  Port=6
  ESC_tiSampling_s : Inport  Port=7
  EvpMod_HtFlwPostReac : Subsystem
  EvpMod_HtFlwPreReac : Subsystem
  EvpMod_InSigHdl : Subsystem
  EvpMod_UCatUsTEst : Subsystem
  EvpMod_tUCatUsT : Outport
  EvpMod_tUCatDsT : Outport  Port=2
  wires:
  EvpMod_InSigHdl/1(dmRdcAgCnv) -> EvpMod_HtFlwPreReac/1(dmRdcAgCnv)
  EvpMod_InSigHdl/2(dmWtVapo) -> EvpMod_HtFlwPostReac/2(dmWtVapo), EvpMod_HtFlwPreReac/4(dmWtVapo)
  EvpMod_InSigHdl/3(dmUrea) -> EvpMod_HtFlwPostReac/1(dmUrea), EvpMod_HtFlwPreReac/5(dmUrea)
  SCRT_tUCatDsT/1 -> EvpMod_tUCatDsT/1
  EvpMod_HtFlwPostReac/4(dwCO2) -> EvpMod_UCatUsTEst/8(dwCO2)
  EvpMod_HtFlwPostReac/3(dwNH3) -> EvpMod_UCatUsTEst/7(dwNH3)
  EvpMod_HtFlwPreReac/1(dwRdcAg) -> EvpMod_UCatUsTEst/1(dwRdcAg)
  EvpMod_HtFlwPreReac/2(dwPhChngWt) -> EvpMod_UCatUsTEst/2(dwPhChngWt)
  EvpMod_HtFlwPreReac/3(dwUrea) -> EvpMod_UCatUsTEst/3(dwUrea)
  EvpMod_HtFlwPreReac/4(dwWtPreReac) -> EvpMod_UCatUsTEst/4(dwWtPreReac)
  EvpMod_HtFlwPostReac/1(dwUreaReac) -> EvpMod_UCatUsTEst/5(dwUreaReac)
  EvpMod_HtFlwPostReac/2(dwWtPostReac) -> EvpMod_UCatUsTEst/6(dwWtPostReac)
  EvpMod_InSigHdl/4(dmEG) -> EvpMod_UCatUsTEst/10(dmEG)
  EvpMod_InSigHdl/5(cpRdcAg) -> EvpMod_HtFlwPreReac/2(cpRdcAg)
  EvpMod_InSigHdl/6(cpUrea) -> EvpMod_HtFlwPreReac/6(cpUrea)
  EvpMod_InSigHdl/7(cpWtPreReac) -> EvpMod_HtFlwPreReac/7(cpWtPreReac)
  EvpMod_InSigHdl/9(cpNH3) -> EvpMod_HtFlwPostReac/5(cpNH3)
  EvpMod_InSigHdl/10(cpCO2) -> EvpMod_HtFlwPostReac/6(cpCO2)
  EvpMod_InSigHdl/11(cpEG) -> EvpMod_UCatUsTEst/11(cpEG)
  EvpMod_InSigHdl/8(cpWtPostReac) -> EvpMod_HtFlwPostReac/3(cpWtPostReac)
  EvpMod_UCatUsTEst/1(tUCatUsTEst) -> EvpMod_tUCatUsT/1
  SCR_tUCatUsT/1 -> EvpMod_InSigHdl/4(tUCatUsT), EvpMod_UCatUsTEst/9(tUCatUsT), EvpMod_HtFlwPostReac/4(tUCatUsT)
  ASMod_dmEGFld/1 -> EvpMod_InSigHdl/3(dmEGFId)
  SCR_tUTnkT/1 -> EvpMod_InSigHdl/5(tUTnkT), EvpMod_HtFlwPreReac/3(tUTnkT)
  UDC_dmRdcAgDes/1 -> EvpMod_InSigHdl/2(dmRdcAgDes)
  UDC_dmRdcAgAct/1 -> EvpMod_InSigHdl/1(dmRdcAgAct)
  ESC_tiSampling_s/1 -> EvpMod_UCatUsTEst/12(tiSampling)

== system Virtual_Exhaust_Aftertreatment_Controller_PRT/UCatCtrl/Urea_Dosing_Control/Feed Forward Dosing ==
  ATS_rNOxUCatUs_ppm : Inport
  ATS_etaEstNOxCnvUCat : Inport  Port=2
  ATS_rNO2NOxUCatUs : Inport  Port=3
  ATS_mflEG : Inport  Port=4
  ATS_tEstUCatAvrg : Inport  Port=5
  ATS_facEffUCatAge : Inport  Port=6
  ATS_mflNH3OxiUCatUs_mgps : Inport  Port=7
  Add2 : Sum
  Constant1 : Constant  Value=3.6  SampleTime=-1
  Constant2 : Constant  Value=46/29  SampleTime=-1
  Constant3 : Constant  Value=1000  SampleTime=-1
  Constant4 : Constant  Value=1e6  SampleTime=-1
  Constant_1 : Constant  SampleTime=-1
  Divide : Product  Inputs=*/
  Divide2 : Product  Inputs=*/
  Interpolation Using Prelookup : Interpolation_n-D  NumberOfTableDimensions=1  TableSource=Input port  Table=|  ExtrapMethod=Clip  ValidIndexMayReachLast=on
      | [    0.2790    0.2970    0.3080    0.3220    0.3510    0.4240    0.5640    0.6550    0.8190    1.0000    1.0000    1.0000
      |     0.3260    0.3430    0.3540    0.3670    0.3960    0.4660    0.6010    0.6900    0.8440    1.0000    1.0000    1.0000
      |     0.3730    0.3890    0.4000    0.4130    0.4400    0.5080    0.6380    0.7230    0.8680    1.0000    1.0000    1.0000
      |     0.4320    0.4480    0.4580    0.4700    0.4960    0.5600    0.6830    0.7640    0.8970    1.0000    1.0000    1.0000
      |     0.4920    0.5070    0.5160    0.5270    0.5520    0.6120    0.7260    0.8020    0.9220    1.0000    1.0000    1.0000
      |     0.5510    0.5650    0.5730    0.5840    0.6070    0.6620    0.7680    0.8370    0.9410    1.0000    1.0000    1.0000
      |     0.6070    0.6200    0.6280    0.6380    0.6600    0.7130    0.8130    0.8750    0.9580    1.0000    1.0000    1.0000
      |     0.6580    0.6710    0.6790    0.6890    0.7110    0.7630    0.8600    0.9130    0.9730    1.0000    1.0000    1.0000
      |     0.7030    0.7170    0.7250    0.7360    0.7580    0.8130    0.9110    0.9540    0.9900    1.0000    1.0000    1.0000
      |     0.7620    0.7790    0.7900    0.8030    0.8300    0.8980    1.0000    1.0000    1.0000    1.0000    1.0000    1.0000
      |     0.7840    0.7980    0.8060    0.8160    0.8370    0.8910    0.9920    1.0000    1.0000    1.0000    1.0000    1.0000
      |     0.7800    0.8780    0.8820    0.8860    0.8950    0.9180    0.9620    1.0000    1.0000    1.0000    1.0000    1.0000
      | ]
      settings: InputPortMap=u0,u1,p2
  Lookup_n-D_3 : Lookup_n-D  BreakpointsForDimension1=[-0.0400000000000091;129.96;149.96;349.96;374.96;424.96;449.96;499.96;549.96;599.96;649.96;699.96]  BreakpointsForDimension2=[0 0.09 0.18 0.27 0.36 0.45 0.54 0.63 0.72 0.81 0.91 1]  Table=[0.375 0.375 0.375 0.375 0.375 0.375 0.375 0.375 0.375 0.375 0.375 0.375;0.375 0.375 0.375 0.375 0.375 0.375 0.375 0.375 0.375 0.375 0.375 0.375;0.375 0.375 0.375 0.375 0.375 0.375 0.375 0.375 0.375 0.375 0.375 0.375;0.379 0.379 0.379 0.379 0.379 0.379 0.379 0.379 0.379 0.379 0.379 0.379;0.379 0.379 0.379 0.379 0.379 0.379 0.379 0.379 0.379 0.379 0.379 0.379;0.383 0.383 0.383 0.383 0.383 0.383 0.383 0.383 0.383 0.383 0.383 0.383;0.461 0.461 0.461 0.461 0.461 0.461 0.461 0.461 0.461 0.461 0.461 0.461;0.48 0.48 0.48 0.48 0.48 0.48 0.48 0.48 0.48 0.48 0.48 0.48;0.738 0.738 0.738 0.738 0.738 0.738 0.738 0.738 0.738 0.738 0.738 0.738;0.923 0.923 0.923 0.923 0.923 0.923 0.923 0.923 0.923 0.923 0.923 0.923;0.923 0.923 0.923 0.923 0.923 0.923 0.923 0.923 0.923 0.923 0.923 0.923;0.923 0.923 0.923 0.923 0.923 0.923 0.923 0.923 0.923 0.923 0.923 0.923]  ExtrapMethod=Clip  UseLastTableValue=on  RndMeth=Simplest  InputSameDT=on
  Lookup_n-D_4 : Lookup_n-D  BreakpointsForDimension1=[-0.0400000000000091;129.96;149.96;349.96;374.96;424.96;449.96;499.96;549.96;599.96;649.96;699.96]  BreakpointsForDimension2=[0 0.09 0.18 0.27 0.36 0.45 0.54 0.63 0.72 0.81 0.91 1]  Table=[0.375 0.375 0.375 0.375 0.375 0.375 0.375 0.375 0.375 0.375 0.375 0.375;0.375 0.375 0.375 0.375 0.375 0.375 0.375 0.375 0.375 0.375 0.375 0.375;0.375 0.375 0.375 0.375 0.375 0.375 0.375 0.375 0.375 0.375 0.375 0.375;0.379 0.379 0.379 0.379 0.379 0.379 0.379 0.379 0.379 0.379 0.379 0.379;0.379 0.379 0.379 0.379 0.379 0.379 0.379 0.379 0.379 0.379 0.379 0.379;0.383 0.383 0.383 0.383 0.383 0.383 0.383 0.383 0.383 0.383 0.383 0.383;0.461 0.461 0.461 0.461 0.461 0.461 0.461 0.461 0.461 0.461 0.461 0.461;0.48 0.48 0.48 0.48 0.48 0.48 0.48 0.48 0.48 0.48 0.48 0.48;0.738 0.738 0.738 0.738 0.738 0.738 0.738 0.738 0.738 0.738 0.738 0.738;0.923 0.923 0.923 0.923 0.923 0.923 0.923 0.923 0.923 0.923 0.923 0.923;0.923 0.923 0.923 0.923 0.923 0.923 0.923 0.923 0.923 0.923 0.923 0.923;0.923 0.923 0.923 0.923 0.923 0.923 0.923 0.923 0.923 0.923 0.923 0.923]  ExtrapMethod=Clip  UseLastTableValue=on  RndMeth=Simplest  InputSameDT=on
  Multiport Switch : MultiPortSwitch  DataPortOrder=Zero-based contiguous  Inputs=2
  Mux1 : Mux  Inputs=2
  Prelookup : PreLookup  BreakpointsData=[0 1]  UseLastBreakpoint=on
  Product1 : Product  Inputs=4  RndMeth=Zero
  Product2 : Product  RndMeth=Zero
  Product3 : Product  RndMeth=Zero
  ATS_mflNH3Cnv_mgps : Outport
  ATS_mflNOxUs_mgps : Outport  Port=2
  ATS_mflNH3PreCtl_mgps : Outport  Port=3
  wires:
  ATS_mflEG/1 -> Divide/1
  Constant1/1 -> Divide/2
  Divide/1 -> Product1/2
  ATS_rNOxUCatUs_ppm/1 -> Product1/1
  Constant2/1 -> Product1/3
  Constant3/1 -> Product1/4
  Constant4/1 -> Divide2/2
  Divide2/1 -> ATS_mflNOxUs_mgps/1, Product2/1
  ATS_tEstUCatAvrg/1 -> Lookup_n-D_4/1, Lookup_n-D_3/1
  Lookup_n-D_3/1 -> Mux1/1
  Lookup_n-D_4/1 -> Mux1/2
  Interpolation Using Prelookup/1 -> Product2/2
  Prelookup/1 -> Interpolation Using Prelookup/1
  Prelookup/2 -> Interpolation Using Prelookup/2
  ATS_rNO2NOxUCatUs/1 -> Lookup_n-D_4/2, Lookup_n-D_3/2
  Product2/1 -> Product3/1
  Product3/1 -> Add2/2, Multiport Switch/2, ATS_mflNH3Cnv_mgps/1
  Product1/1 -> Divide2/1
  Mux1/1 -> Interpolation Using Prelookup/3
  ATS_facEffUCatAge/1 -> Prelookup/1
  ATS_etaEstNOxCnvUCat/1 -> Product3/2
  Add2/1 -> Multiport Switch/3
  Constant_1/1 -> Multiport Switch/1
  Multiport Switch/1 -> ATS_mflNH3PreCtl_mgps/1
  ATS_mflNH3OxiUCatUs_mgps/1 -> Add2/1
